simulink model "sla_VHT_HDL"  (R2015a)
settings: Solver=FixedStepDiscrete  SolverMode=SingleTasking  StartTime=0.0  StopTime=320*240*100  RelTol=1e-3
undefined symbols (not defined in the file): gray, H
libraries: visionsinks x3, visionhdlio x2, visionhdlconversions x1, visionhdlfilter x1, visionconversions x1, dspvision x1
settings Model: SimulationMode=accelerator  CovSFcnEnable=off  Creator=yutengz  LastModifiedBy=amatsumo
settings OptimizationCC: BlockReduction=off  BooleanDataType=off
settings DebuggingCC: SaveWithParameterizedLinksMsg=none  UnderspecifiedInitializationDetection=Classic  MergeDetectMultiDrivingBlocksExec=none  SignalResolutionControl=TryResolveAllWithWarning
settings HardwareCC: TargetUnknown=on

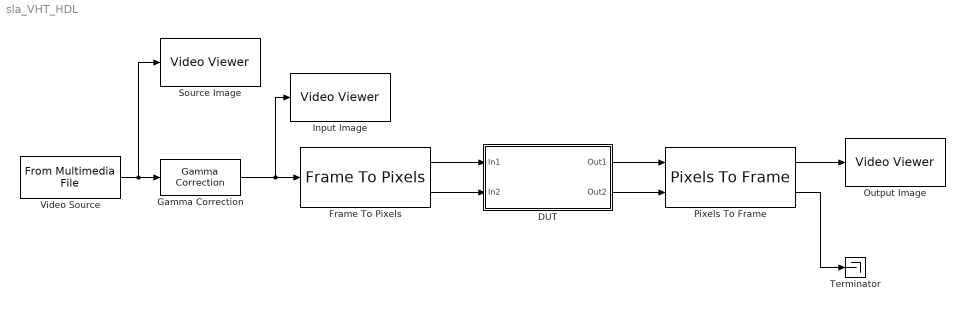
== system sla_VHT_HDL ==
  DUT : Subsystem
  Frame To Pixels : visionhdlio/Frame To Pixels  NumComponents=1  VideoFormat=240p  ActivePixelsPerLine=32  ActiveVideoLines=18  TotalPixelsPerLine=42  TotalVideoLines=28  StartingActiveLine=6  FrontPorch=5  SampleTime=0
  Gamma Correction : visionconversions/Gamma Correction  operation=De-gamma  gamma=2.2  linearSegment=on  breakPoint=0.018
  Input Image : visionsinks/Video Viewer  inputType=Obsolete7b  imagePorts=One multidimensional signal  useColorMap=off  colormapValue=gray(256)  specRange=off  minInputVal=0  maxInputVal=255  FigPos=[366 381 334 275]  AxisZoom=on  trueSizedOnce=off  OpenAtMdlStart=on  DefaultConfigurationName=vipscopes.VideoViewerScopeCfg
  Output Image : visionsinks/Video Viewer  inputType=Obsolete7b  imagePorts=One multidimensional signal  useColorMap=off  colormapValue=gray(256)  specRange=off  minInputVal=0  maxInputVal=255  FigPos=[709 384 334 275]  AxisZoom=on  trueSizedOnce=off  OpenAtMdlStart=on  DefaultConfigurationName=vipscopes.VideoViewerScopeCfg
  Pixels To Frame : visionhdlio/Pixels To Frame  NumComponents=1  VideoFormat=240p  ActivePixelsPerLine=32  ActiveVideoLines=18  TotalPixelsPerLine=42  TotalVideoLines=28
  Source Image : visionsinks/Video Viewer  inputType=Obsolete7b  imagePorts=One multidimensional signal  useColorMap=off  colormapValue=gray(256)  specRange=off  minInputVal=0  maxInputVal=255  FigPos=[21 379 334 275]  AxisZoom=on  trueSizedOnce=off  OpenAtMdlStart=on  DefaultConfigurationName=vipscopes.VideoViewerScopeCfg
  Terminator : Terminator
  Video Source : dspvision/From Multimedia File  inputFilename=rhinos.avi  loop=on  numPlays=inf  outputStreams=Video only  videoDataType=uint8  audioDataType=int16  inheritSampleTime=off  userDefinedSampleTime=402*324  noAudioOutput=off  isIntensityVideo=off  fourcc=Intensity  colorVideoFormat=One multidimensional signal  outputEOF=off  dataOrg=Column-major  audioFrameSize=1024  computeAudioFrameSize=off  outSamplingMode=Sample based
  wires:
  Video Source/1 -> Source Image/1, Gamma Correction/1
  Pixels To Frame/1 -> Output Image/1
  Pixels To Frame/2 -> Terminator/1
  Gamma Correction/1 -> Input Image/1, Frame To Pixels/1
  Frame To Pixels/1 -> DUT/1(In1)
  Frame To Pixels/2 -> DUT/2(In2)
  DUT/1(Out1) -> Pixels To Frame/1
  DUT/2(Out2) -> Pixels To Frame/2

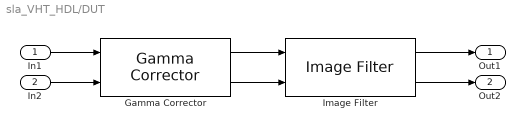
== system sla_VHT_HDL/DUT ==
  In1 : Inport
  In2 : Inport  Port=2
  Gamma Corrector : visionhdlconversions/Gamma Corrector  Correction=Gamma  Gamma=2.2  LinearSegment=on  BreakPoint=0.018  SimulateUsing=Code generation
  Image Filter : visionhdlfilter/Image Filter  Coefficients=H  PaddingMethod=Replicate  PaddingValue=0  LineBufferSize=2048  roundingMode=Floor  overflowMode=on  CoeffDataTypeStr=fixdt(1,8,4)  CoeffMin=[]  CoeffMax=[]  OutputMin=[]  OutputMax=[]  SimulateUsing=Code generation
  Out1 : Outport
  Out2 : Outport  Port=2
  wires:
  In2/1 -> Gamma Corrector/2
  Gamma Corrector/2 -> Image Filter/2
  In1/1 -> Gamma Corrector/1
  Image Filter/2 -> Out2/1
  Gamma Corrector/1 -> Image Filter/1
  Image Filter/1 -> Out1/1
